simulink model "PresaDepredador_ejm2"  (R2020a)
settings: Solver=ode45  StartTime=0.0  StopTime=Time  RelTol=1e-3
undefined symbols (not defined in the file): alpha, beta, D0, delta, gamma, P0
settings Model: Creator=mluser  LastModifiedBy=curie
settings DataIOCC: ReturnWorkspaceOutputs=off

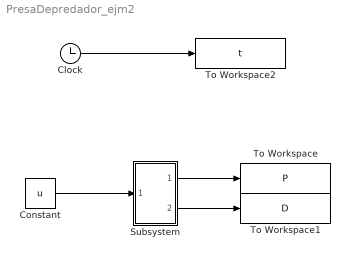
== system PresaDepredador_ejm2 ==
  Clock : Clock
  Constant : Constant  Value=u
  Subsystem : Subsystem
  To Workspace : ToWorkspace  VariableName=P  SampleTime=-1
      settings: Save2DSignal=2-D array (concatenate along first dimension)
  To Workspace1 : ToWorkspace  VariableName=D  SampleTime=-1
      settings: Save2DSignal=2-D array (concatenate along first dimension)
  To Workspace2 : ToWorkspace  VariableName=t  SampleTime=-1
      settings: Save2DSignal=2-D array (concatenate along first dimension)
  wires:
  Clock/1 -> To Workspace2/1
  Constant/1 -> Subsystem/1(In1)
  Subsystem/1(Out1) -> To Workspace/1
  Subsystem/2(Out2) -> To Workspace1/1

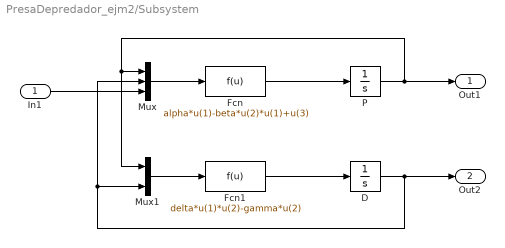
== system PresaDepredador_ejm2/Subsystem ==
  In1 : Inport
  D : Integrator  InitialCondition=D0
  Fcn : Fcn  Expr=alpha*u(1)-beta*u(2)*u(1)+u(3)
  Fcn1 : Fcn  Expr=delta*u(1)*u(2)-gamma*u(2)
  Mux : Mux  Inputs=3
  Mux1 : Mux  Inputs=2
  P : Integrator  InitialCondition=P0
  Out1 : Outport
  Out2 : Outport  Port=2
  wires:
  Mux/1 -> Fcn/1
  Mux1/1 -> Fcn1/1
  Fcn/1 -> P/1
  D/1 -> Out2/1, Mux1/2, Mux/2
  P/1 -> Out1/1, Mux1/1, Mux/1
  In1/1 -> Mux/3
  Fcn1/1 -> D/1
